simulink model "gtm_aeromodel"  (Simulink 7.2)
settings: Solver=ode45  StartTime=0.0  StopTime=10.0  RelTol=1e-3
undefined symbols (not defined in the file or in its folder): A_BLCG, A_BW, A_CW, A_FSCG, A_FSREF_in, A_SW, A_WLCG, A_WLREF, ALPHA0, bclowb, bclowbx_FMACH, bcmowb, bcmowbx_FHP, bcmowby_FMACH, cda, cdax_FLPDEF, cddr, cddrx_FMACH, cdo, cdox_FLPDEF, cdt1, cdt1x_mach, cdt2, cdt2x_mach, cdto, cdtox_mach, cdwb, cdwbx_FALPHA, cdwby_FMACH, clat, clatfr, clatfrx_FHP, clatfry_FMACH, clatx_mach, clawbfr, clawbfrx_FHP, clawbfry_FMACH, cldefr, cldefrx_FHP, cldefry_FMACH, cldtab, cldtabx_FMACH, clqwb, clqwbfr, clqwbfrx_FHP, clqwbfry_FMACH, clqwbx_mach, cltdd, cltddx_FHP, cltddy_FMACH, clwb, clwbtdd, clwbtddx_FHP, clwbtddy_FMACH, clwbx_FALPHA, clwby_FMACH, clwbzdd, clwbzddx_FHP, clwbzddy_FMACH, clzdd ... (+196)
libraries: model_lib x1
(part 2 of 10)

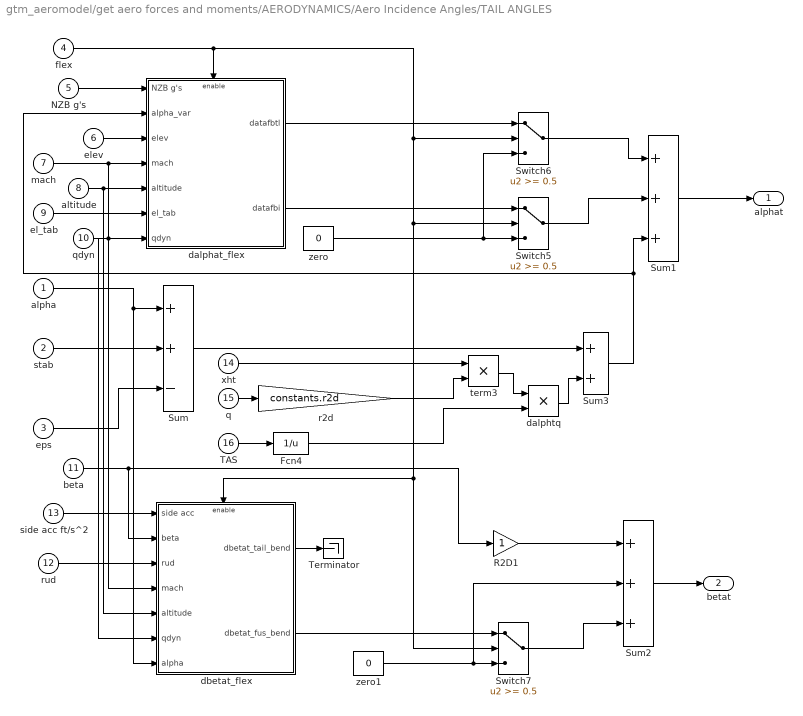
== system gtm_aeromodel/get aero forces and moments/AERODYNAMICS/Aero Incidence Angles/TAIL ANGLES ==
  alpha : Inport  OutDataType=sfix(16)  OutScaling=2^0
  stab : Inport  Port=2  OutDataType=sfix(16)  OutScaling=2^0
  eps : Inport  Port=3  OutDataType=sfix(16)  OutScaling=2^0
  flex : Inport  Port=4  OutDataType=sfix(16)  OutScaling=2^0
  NZB g's : Inport  Port=5  OutDataType=sfix(16)  OutScaling=2^0
  elev : Inport  Port=6  OutDataType=sfix(16)  OutScaling=2^0
  mach : Inport  Port=7  OutDataType=sfix(16)  OutScaling=2^0
  altitude : Inport  Port=8  OutDataType=sfix(16)  OutScaling=2^0
  el_tab : Inport  Port=9  OutDataType=sfix(16)  OutScaling=2^0
  qdyn : Inport  Port=10  OutDataType=sfix(16)  OutScaling=2^0
  beta : Inport  Port=11  OutDataType=sfix(16)  OutScaling=2^0
  rud : Inport  Port=12  OutDataType=sfix(16)  OutScaling=2^0
  side acc ft/s^2 : Inport  Port=13  OutDataType=sfix(16)  OutScaling=2^0
  xht : Inport  Port=14  OutDataType=sfix(16)  OutScaling=2^0
  q : Inport  Port=15  OutDataType=sfix(16)  OutScaling=2^0
  TAS : Inport  Port=16  OutDataType=sfix(16)  OutScaling=2^0
  Fcn4 : Fcn  Expr=1/u
  R2D1 : Gain  ParameterDataType=sfix(16)  ParameterScaling=2^0  OutDataType=sfix(16)  OutScaling=2^0  SaturateOnIntegerOverflow=on  OutDataTypeStr=Inherit: Same as input  ParamDataTypeStr=Inherit: Same as input
  Sum : Sum  Inputs=++-  OutDataType=sfix(16)  OutScaling=2^0  SaturateOnIntegerOverflow=on  InputSameDT=on  OutDataTypeStr=Inherit: Same as first input
  Sum1 : Sum  Inputs=+++  OutDataType=sfix(16)  OutScaling=2^0  SaturateOnIntegerOverflow=on  InputSameDT=on  OutDataTypeStr=Inherit: Same as first input
  Sum2 : Sum  Inputs=+++  OutDataType=sfix(16)  OutScaling=2^0  SaturateOnIntegerOverflow=on  InputSameDT=on  OutDataTypeStr=Inherit: Same as first input
  Sum3 : Sum  OutDataType=sfix(16)  OutScaling=2^0  SaturateOnIntegerOverflow=on  InputSameDT=on  OutDataTypeStr=Inherit: Same as first input
  Switch5 : Switch  Threshold=0.5  SaturateOnIntegerOverflow=on  InputSameDT=on
  Switch6 : Switch  Threshold=0.5  SaturateOnIntegerOverflow=on  InputSameDT=on
  Switch7 : Switch  Threshold=0.5  SaturateOnIntegerOverflow=on  InputSameDT=on
  Terminator : Terminator
  dalphat_flex : Subsystem  TreatAsAtomicUnit=on
  dalphtq : Product  OutDataType=sfix(16)  OutScaling=2^0  SaturateOnIntegerOverflow=on  RndMeth=Zero  InputSameDT=on  OutDataTypeStr=Inherit: Same as first input
  dbetat_flex : Subsystem  TreatAsAtomicUnit=on
  r2d : Gain  Gain=constants.r2d  ParameterDataType=sfix(16)  ParameterScaling=2^0  OutDataType=sfix(16)  OutScaling=2^0  SaturateOnIntegerOverflow=on  OutDataTypeStr=Inherit: Same as input  ParamDataTypeStr=Inherit: Same as input
  term3 : Product  OutDataType=sfix(16)  OutScaling=2^0  SaturateOnIntegerOverflow=on  RndMeth=Zero  InputSameDT=on  OutDataTypeStr=Inherit: Same as first input
  zero : Constant  Value=0  OutDataType=sfix(16)  OutScaling=2^0
  zero1 : Constant  Value=0  OutDataType=sfix(16)  OutScaling=2^0
  alphat : Outport  OutDataType=sfix(16)  OutScaling=2^0
  betat : Outport  Port=2  OutDataType=sfix(16)  OutScaling=2^0
  wires:
  r2d/1 -> term3/2
  q/1 -> r2d/1
  alpha/1 -> Sum/1, dbetat_flex/7(alpha)
  stab/1 -> Sum/2
  eps/1 -> Sum/3
  dalphtq/1 -> Sum3/2
  Switch5/1 -> Sum1/2
  Switch6/1 -> Sum1/1
  R2D1/1 -> Sum2/1
  mach/1 -> dbetat_flex/4(mach), dalphat_flex/4(mach)
  altitude/1 -> dbetat_flex/5(altitude), dalphat_flex/5(altitude)
  qdyn/1 -> dbetat_flex/6(qdyn), dalphat_flex/7(qdyn)
  flex/1 -> dalphat_flex/Enable, dbetat_flex/Enable, Switch7/2, Switch5/2, Switch6/2
  zero/1 -> Switch5/3, Switch6/3
  dalphat_flex/2(datafbi) -> Switch5/1
  NZB g's/1 -> dalphat_flex/1(NZB g's)
  elev/1 -> dalphat_flex/3(elev)
  el_tab/1 -> dalphat_flex/6(el_tab)
  side acc ft/s^2/1 -> dbetat_flex/1("side acc ")
  rud/1 -> dbetat_flex/3(rud)
  beta/1 -> R2D1/1, dbetat_flex/2(beta)
  Sum2/1 -> betat/1
  dbetat_flex/1(dbetat_tail_bend) -> Terminator/1
  xht/1 -> term3/1
  TAS/1 -> Fcn4/1
  term3/1 -> dalphtq/1
  Fcn4/1 -> dalphtq/2
  dalphat_flex/1(datafbtl) -> Switch6/1
  Sum/1 -> Sum3/1
  Sum3/1 -> dalphat_flex/2(alpha_var), Sum1/3
  dbetat_flex/2(dbetat_fus_bend) -> Switch7/1
  Switch7/1 -> Sum2/3
  zero1/1 -> Sum2/2, Switch7/3
  Sum1/1 -> alphat/1

== system gtm_aeromodel/get aero forces and moments/AERODYNAMICS/Force  Coefficients/DRAG  ==
  flex : Inport  OutDataType=sfix(16)  OutScaling=2^0
  ige : Inport  Port=2  OutDataType=sfix(16)  OutScaling=2^0
  hob : Inport  Port=3  OutDataType=sfix(16)  OutScaling=2^0
  alpha : Inport  Port=4  OutDataType=sfix(16)  OutScaling=2^0
  mach : Inport  Port=5  OutDataType=sfix(16)  OutScaling=2^0
  altitude : Inport  Port=6  OutDataType=sfix(16)  OutScaling=2^0
  flap : Inport  Port=7  OutDataType=sfix(16)  OutScaling=2^0
  gear : Inport  Port=8  OutDataType=sfix(16)  OutScaling=2^0
  dsb : Inport  Port=9  OutDataType=sfix(16)  OutScaling=2^0
  dsl : Inport  Port=10  OutDataType=sfix(16)  OutScaling=2^0
  rud : Inport  Port=11  OutDataType=sfix(16)  OutScaling=2^0
  aill : Inport  Port=12  OutDataType=sfix(16)  OutScaling=2^0
  alphat : Inport  Port=13  OutDataType=sfix(16)  OutScaling=2^0
  elev : Inport  Port=14  OutDataType=sfix(16)  OutScaling=2^0
  ailr : Inport  Port=15  OutDataType=sfix(16)  OutScaling=2^0
  dsr : Inport  Port=16  OutDataType=sfix(16)  OutScaling=2^0
  clwb : Inport  Port=17  OutDataType=sfix(16)  OutScaling=2^0
  CDAIL : Subsystem
  CDGE : Subsystem  TreatAsAtomicUnit=on
  CDGEAR : Subsystem
  CDR : Subsystem
  CDSPOIL : Subsystem
  CDTP : Subsystem
  CDWB : Subsystem
  DCDDEL : Subsystem
  Sum1 : Sum  Inputs=+++++  OutDataType=sfix(16)  OutScaling=2^0  SaturateOnIntegerOverflow=on  InputSameDT=on  OutDataTypeStr=Inherit: Same as first input
  Sum8 : Sum  Inputs=++++++++  OutDataType=sfix(16)  OutScaling=2^0  SaturateOnIntegerOverflow=on  InputSameDT=on  OutDataTypeStr=Inherit: Same as first input
  Switch6 : Switch  Threshold=0.5  SaturateOnIntegerOverflow=on  InputSameDT=on
  bcddf : Subsystem  TreatAsAtomicUnit=on
  bcdwb : Subsystem
  constant1 : Constant  Value=0.0  OutDataType=sfix(16)  OutScaling=2^0
  CD8 : Outport  OutDataType=sfix(16)  OutScaling=2^0  InitialOutput=0
  cdtp : Outport  Port=2  OutDataType=sfix(16)  OutScaling=2^0  InitialOutput=0
  dcddel : Outport  Port=3  OutDataType=sfix(16)  OutScaling=2^0  InitialOutput=0
  wires:
  bcddf/1(bcddf) -> Sum8/8
  bcdwb/1(bcdwb_) -> Sum8/7
  DCDDEL/1(dcdde) -> dcddel/1
  CDAIL/1(cdail) -> Sum8/6
  CDTP/1(cdtp) -> cdtp/1
  CDGEAR/1(cdg) -> Sum8/4
  CDR/1(cdrud) -> Sum8/3
  CDSPOIL/3(cd_sp_int_df) -> Sum1/4
  CDSPOIL/2(cd_sb) -> Sum1/3
  CDSPOIL/1(cd_spoil) -> Sum1/2
  CDWB/3(dcdsbfint) -> Sum1/5
  CDWB/2(cd_flap) -> Sum1/1
  CDWB/1(cdwb) -> Sum8/1
  Sum8/1 -> CD8/1
  Sum1/1 -> Sum8/2
  flap/1 -> CDWB/3(flap), CDGEAR/1(flap), CDGE/3(flap), bcddf/1(flap), CDSPOIL/5(flap)
  mach/1 -> CDWB/2(mach), CDR/1(mach), CDTP/1(mach), DCDDEL/3(mach), CDSPOIL/4(mach)
  alpha/1 -> CDWB/1(alpha), CDGEAR/2(alpha), CDGE/2(alpha), CDSPOIL/3(alpha)
  alphat/1 -> CDTP/2(alphat), DCDDEL/2(alphat)
  elev/1 -> DCDDEL/1(elev)
  ailr/1 -> CDAIL/2(ailr)
  hob/1 -> CDGE/1(hob)
  aill/1 -> CDAIL/1(aill)
  constant1/1 -> Switch6/3
  CDGE/1(cdge) -> Switch6/1
  Switch6/1 -> Sum8/5
  ige/1 -> Switch6/2
  rud/1 -> CDR/2(rud)
  gear/1 -> CDGEAR/3(gear)
  dsl/1 -> CDSPOIL/2(dsl)
  dsr/1 -> CDSPOIL/6(dsr)
  altitude/1 -> CDWB/5(altitude)
  flex/1 -> CDWB/4(flex)
  dsb/1 -> CDSPOIL/1(dsb), CDWB/6(dsb)
  clwb/1 -> bcdwb/1(clwb)

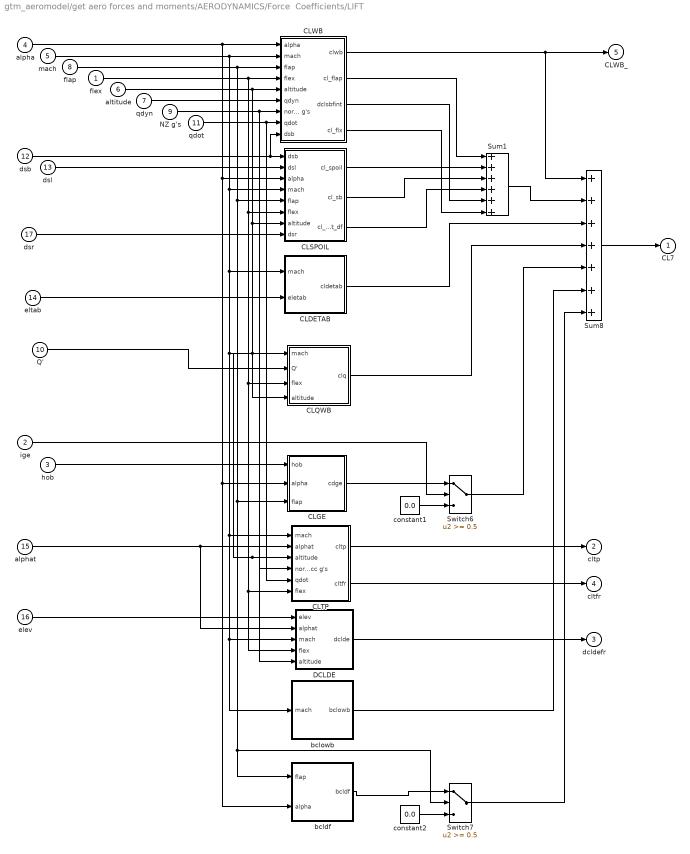
== system gtm_aeromodel/get aero forces and moments/AERODYNAMICS/Force  Coefficients/LIFT ==
  flex : Inport  OutDataType=sfix(16)  OutScaling=2^0
  ige : Inport  Port=2  OutDataType=sfix(16)  OutScaling=2^0
  hob : Inport  Port=3  OutDataType=sfix(16)  OutScaling=2^0
  alpha : Inport  Port=4  OutDataType=sfix(16)  OutScaling=2^0
  mach : Inport  Port=5  OutDataType=sfix(16)  OutScaling=2^0
  altitude : Inport  Port=6  OutDataType=sfix(16)  OutScaling=2^0
  qdyn : Inport  Port=7  OutDataType=sfix(16)  OutScaling=2^0
  flap : Inport  Port=8  OutDataType=sfix(16)  OutScaling=2^0
  NZ g's : Inport  Port=9  OutDataType=sfix(16)  OutScaling=2^0
  Q' : Inport  Port=10  OutDataType=sfix(16)  OutScaling=2^0
  qdot : Inport  Port=11  OutDataType=sfix(16)  OutScaling=2^0
  dsb : Inport  Port=12  OutDataType=sfix(16)  OutScaling=2^0
  dsl : Inport  Port=13  OutDataType=sfix(16)  OutScaling=2^0
  eltab : Inport  Port=14  OutDataType=sfix(16)  OutScaling=2^0
  alphat : Inport  Port=15  OutDataType=sfix(16)  OutScaling=2^0
  elev : Inport  Port=16  OutDataType=sfix(16)  OutScaling=2^0
  dsr : Inport  Port=17  OutDataType=sfix(16)  OutScaling=2^0
  CLDETAB : Subsystem
  CLGE : Subsystem  TreatAsAtomicUnit=on
  CLQWB : Subsystem
  CLSPOIL : Subsystem
  CLTP : Subsystem
  CLWB : Subsystem
  DCLDE : Subsystem
  Sum1 : Sum  Inputs=++++++  OutDataType=sfix(16)  OutScaling=2^0  SaturateOnIntegerOverflow=on  InputSameDT=on  OutDataTypeStr=Inherit: Same as first input
  Sum8 : Sum  Inputs=+++++++  OutDataType=sfix(16)  OutScaling=2^0  SaturateOnIntegerOverflow=on  InputSameDT=on  OutDataTypeStr=Inherit: Same as first input
  Switch6 : Switch  Threshold=0.5  SaturateOnIntegerOverflow=on  InputSameDT=on
  Switch7 : Switch  Threshold=0.5  SaturateOnIntegerOverflow=on  InputSameDT=on
  bcldf : Subsystem  TreatAsAtomicUnit=on
  bclowb : Subsystem
  constant1 : Constant  Value=0.0  OutDataType=sfix(16)  OutScaling=2^0
  constant2 : Constant  Value=0.0  OutDataType=sfix(16)  OutScaling=2^0
  CL7 : Outport  OutDataType=sfix(16)  OutScaling=2^0  InitialOutput=0
  cltp : Outport  Port=2  OutDataType=sfix(16)  OutScaling=2^0  InitialOutput=0
  dcldefr : Outport  Port=3  OutDataType=sfix(16)  OutScaling=2^0  InitialOutput=0
  cltfr : Outport  Port=4  OutDataType=sfix(16)  OutScaling=2^0  InitialOutput=0
  CLWB_ : Outport  Port=5  OutDataType=sfix(16)  OutScaling=2^0  InitialOutput=0
  wires:
  CLWB/4(cl_flx) -> Sum1/6
  CLWB/1(clwb) -> CLWB_/1, Sum8/1
  alpha/1 -> CLSPOIL/3(alpha), CLGE/2(alpha), bcldf/2(alpha), CLWB/1(alpha)
  mach/1 -> CLSPOIL/4(mach), bclowb/1(mach), DCLDE/3(mach), CLTP/1(mach), CLQWB/1(mach), CLDETAB/1(mach), CLWB/2(mach)
  flap/1 -> CLSPOIL/5(flap), CLGE/3(flap), Switch7/2, bcldf/1(flap), CLWB/3(flap)
  altitude/1 -> DCLDE/5(altitude), CLTP/3(altitude), CLQWB/4(altitude), CLSPOIL/7(altitude), CLWB/5(altitude)
  qdot/1 -> CLTP/5(qdot), CLWB/8(qdot)
  NZ g's/1 -> CLTP/4(norm acc g's), CLWB/7(norm acc g's)
  qdyn/1 -> CLWB/6(qdyn)
  flex/1 -> CLQWB/3(flex), DCLDE/4(flex), CLTP/6(flex), CLSPOIL/6(flex), CLWB/4(flex)
  Switch7/1 -> Sum8/7
  bclowb/1(bclowb) -> Sum8/6
  CLTP/1(cltp) -> cltp/1
  DCLDE/1(dclde) -> dcldefr/1
  CLTP/2(cltfr) -> cltfr/1
  CLQWB/1(clq) -> Sum8/4
  CLSPOIL/3(cl_sp_int_df) -> Sum1/4
  CLDETAB/1(cldetab) -> Sum8/3
  CLSPOIL/2(cl_sb) -> Sum1/3
  CLSPOIL/1(cl_spoil) -> Sum1/2
  CLWB/3(dclsbfint) -> Sum1/5
  CLWB/2(cl_flap) -> Sum1/1
  dsb/1 -> CLWB/9(dsb), CLSPOIL/1(dsb)
  dsr/1 -> CLSPOIL/8(dsr)
  hob/1 -> CLGE/1(hob)
  ige/1 -> Switch6/2
  CLGE/1(cdge) -> Switch6/1
  Switch6/1 -> Sum8/5
  elev/1 -> DCLDE/1(elev)
  alphat/1 -> DCLDE/2(alphat), CLTP/2(alphat)
  eltab/1 -> CLDETAB/2(eletab)
  dsl/1 -> CLSPOIL/2(dsl)
  Sum8/1 -> CL7/1
  Sum1/1 -> Sum8/2
  constant1/1 -> Switch6/3
  constant2/1 -> Switch7/3
  bcldf/1(bcldf) -> Switch7/1
  Q'/1 -> CLQWB/2(Q')

== system gtm_aeromodel/get aero forces and moments/AERODYNAMICS/Force  Coefficients/SIDE ==
  note: dcyt
  flex : Inport  OutDataType=sfix(16)  OutScaling=2^0
  alpha : Inport  Port=2  OutDataType=sfix(16)  OutScaling=2^0
  mach : Inport  Port=3  OutDataType=sfix(16)  OutScaling=2^0
  altitude : Inport  Port=4  OutDataType=sfix(16)  OutScaling=2^0
  flap : Inport  Port=5  OutDataType=sfix(16)  OutScaling=2^0
  gear : Inport  Port=6  OutDataType=sfix(16)  OutScaling=2^0
  dsb : Inport  Port=7  OutDataType=sfix(16)  OutScaling=2^0
  dsl : Inport  Port=8  OutDataType=sfix(16)  OutScaling=2^0
  rud : Inport  Port=9  OutDataType=sfix(16)  OutScaling=2^0
  beta : Inport  Port=10  OutDataType=sfix(16)  OutScaling=2^0
  betat : Inport  Port=11  OutDataType=sfix(16)  OutScaling=2^0
  p_prime : Inport  Port=12  OutDataType=sfix(16)  OutScaling=2^0
  r_prime : Inport  Port=13  OutDataType=sfix(16)  OutScaling=2^0
  dsr : Inport  Port=14  OutDataType=sfix(16)  OutScaling=2^0
  " " : Product  Inputs=3  OutDataType=sfix(16)  OutScaling=2^0  SaturateOnIntegerOverflow=on  RndMeth=Zero  InputSameDT=on  OutDataTypeStr=Inherit: Same as first input
  CYBWB : Subsystem
  CYGEAR : Subsystem
  CYP : Subsystem
  CYR : Subsystem
  CYRUD : Subsystem
  CYSPOIL : Subsystem
  Sum8 : Sum  Inputs=+++++++  OutDataType=sfix(16)  OutScaling=2^0  SaturateOnIntegerOverflow=on  InputSameDT=on  OutDataTypeStr=Inherit: Same as first input
  Switch5 : Switch  Threshold=0.1  SaturateOnIntegerOverflow=on  InputSameDT=on
  TAIL : Subsystem
  constant : Constant  OutDataType=sfix(16)  OutScaling=2^0
  cybwb : Product  Inputs=3  OutDataType=sfix(16)  OutScaling=2^0  SaturateOnIntegerOverflow=on  RndMeth=Zero  InputSameDT=on  OutDataTypeStr=Inherit: Same as first input
  CYS : Outport  OutDataType=sfix(16)  OutScaling=2^0  InitialOutput=0
  wires:
  CYGEAR/1(cdg) -> Sum8/7
  CYR/1(dcyrhat) -> Sum8/6
  CYP/1(dcyphat) -> Sum8/5
  CYSPOIL/1(cy_spoil) -> Sum8/3
  " "/1 -> Sum8/2
  cybwb/1 -> Sum8/1
  beta/1 -> CYGEAR/4(beta), cybwb/3
  gear/1 -> CYGEAR/3(gear)
  r_prime/1 -> CYR/5(r_prime)
  p_prime/1 -> CYP/5(p_prime)
  altitude/1 -> CYR/3(altitude), CYP/3(altitude), CYRUD/3(altitude), CYBWB/5(altitude)
  rud/1 -> CYRUD/2(rud)
  flap/1 -> CYGEAR/1(flap), CYSPOIL/5(flap), CYBWB/3(flap)
  TAIL/1(cyb_ht_vt) -> " "/2
  alpha/1 -> CYGEAR/2(alpha), CYR/2(alpha), CYP/2(alpha), CYSPOIL/3(alpha), TAIL/2(alpha), CYBWB/1(alpha)
  mach/1 -> CYR/1(mach), CYP/1(mach), CYRUD/1(mach), CYSPOIL/4(mach), TAIL/1(mach), CYBWB/2(mach)
  flex/1 -> CYR/4(flex), CYP/4(flex), CYRUD/4(flex), Switch5/2, CYBWB/4(flex)
  betat/1 -> " "/3
  Switch5/1 -> " "/1, cybwb/2
  CYBWB/2(cybfr) -> Switch5/1
  constant/1 -> Switch5/3
  Sum8/1 -> CYS/1
  dsb/1 -> CYSPOIL/1(dsb)
  dsl/1 -> CYSPOIL/2(dsl)
  dsr/1 -> CYSPOIL/6(dsr)
  CYBWB/1(cywb+fl) -> cybwb/1
  CYRUD/1(cyrud) -> Sum8/4

== system gtm_aeromodel/get aero forces and moments/AERODYNAMICS/Moment Coefficients/PITCH ==
  flex : Inport  OutDataType=sfix(16)  OutScaling=2^0
  alpha : Inport  Port=2  OutDataType=sfix(16)  OutScaling=2^0
  mach : Inport  Port=3  OutDataType=sfix(16)  OutScaling=2^0
  altitude : Inport  Port=4  OutDataType=sfix(16)  OutScaling=2^0
  qdyn : Inport  Port=5  OutDataType=sfix(16)  OutScaling=2^0
  flap : Inport  Port=6  OutDataType=sfix(16)  OutScaling=2^0
  dsb : Inport  Port=7  OutDataType=sfix(16)  OutScaling=2^0
  dsl : Inport  Port=8  OutDataType=sfix(16)  OutScaling=2^0
  NZ g's : Inport  Port=9  OutDataType=sfix(16)  OutScaling=2^0
  qdot : Inport  Port=10  OutDataType=sfix(16)  OutScaling=2^0
  qhat : Inport  Port=11  OutDataType=sfix(16)  OutScaling=2^0
  eltab : Inport  Port=12  OutDataType=sfix(16)  OutScaling=2^0
  alphat : Inport  Port=13  OutDataType=sfix(16)  OutScaling=2^0
  elev : Inport  Port=14  OutDataType=sfix(16)  OutScaling=2^0
  dsr : Inport  Port=15  OutDataType=sfix(16)  OutScaling=2^0
  BCMOWB : Subsystem
  CMQWB : Subsystem
  CMSPOIL : Subsystem
  CMT : Subsystem
  CMTAB : Subsystem
  CMWB : Subsystem
  DCMDE : Subsystem
  Look-Up Table : Lookup  InputValues="[0  200  350]"  Table=[1 0.76 0.7]  OutDataType=sfix(16)  OutScaling=2^0  SaturateOnIntegerOverflow=on
  Product : Product  OutDataType=sfix(16)  OutScaling=2^0  SaturateOnIntegerOverflow=on  RndMeth=Zero  InputSameDT=on  OutDataTypeStr=Inherit: Same as first input
  Sum1 : Sum  Inputs=++++++  OutDataType=sfix(16)  OutScaling=2^0  SaturateOnIntegerOverflow=on  InputSameDT=on  OutDataTypeStr=Inherit: Same as first input
  Sum8 : Sum  Inputs=++++++++  OutDataType=sfix(16)  OutScaling=2^0  SaturateOnIntegerOverflow=on  InputSameDT=on  OutDataTypeStr=Inherit: Same as first input
  bcmdf : Subsystem  TreatAsAtomicUnit=on
  CMS : Outport  OutDataType=sfix(16)  OutScaling=2^0  InitialOutput=0
  CMDE : Outport  Port=2  OutDataType=sfix(16)  OutScaling=2^0  InitialOutput=0
  wires:
  bcmdf/1(bcmdf) -> Sum8/8
  BCMOWB/1(bcmowb) -> Sum8/7
  CMT/1(cmt) -> Sum8/5
  CMQWB/1(dcmqwb) -> Sum8/4
  CMTAB/1(cmtab) -> Sum8/3
  CMSPOIL/3(dcmspfint) -> Sum1/4
  CMSPOIL/2(cm_sb) -> Sum1/3
  CMSPOIL/1(cm_spoil) -> Sum1/2
  CMWB/2(cm_flap) -> Sum1/1
  CMWB/3(dcmsbfint) -> Sum1/5
  CMWB/1(cmwb) -> Sum8/1
  Sum8/1 -> CMS/1
  Sum1/1 -> Sum8/2
  flex/1 -> CMSPOIL/6(flex), CMQWB/3(flex), CMT/6(flex), DCMDE/4(flex), CMTAB/4(flex), CMWB/4(flex)
  qdyn/1 -> CMWB/6(qdyn), Look-Up Table/1
  flap/1 -> CMWB/3(flap), CMSPOIL/5(flap), bcmdf/1(flap)
  mach/1 -> CMTAB/1(mach), CMQWB/1(mach), CMT/1(mach), DCMDE/3(mach), BCMOWB/1(mach), CMSPOIL/4(mach), CMWB/2(mach)
  alpha/1 -> CMWB/1(alpha), CMSPOIL/3(alpha), bcmdf/2(alpha)
  dsl/1 -> CMSPOIL/2(dsl)
  qdot/1 -> CMWB/8(qdot), CMT/5(qdot)
  elev/1 -> DCMDE/1(elev)
  qhat/1 -> CMQWB/2(qhat)
  eltab/1 -> CMTAB/2(eletab)
  dsb/1 -> CMSPOIL/1(dsb), CMWB/9(dsb)
  dsr/1 -> CMSPOIL/8(dsr)
  NZ g's/1 -> CMWB/7(norm acc g's), CMT/4(norm acc g's)
  altitude/1 -> CMWB/5(altitude), CMSPOIL/7(altitude), CMTAB/3(alt), CMQWB/4(altitude), CMT/3(altitude), DCMDE/5(altitude), BCMOWB/2(altitude)
  CMWB/4(cm_flx) -> Sum1/6
  alphat/1 -> CMT/2(alphat), DCMDE/2(alphat)
  Look-Up Table/1 -> Product/2
  DCMDE/1(dcmde) -> Product/1
  Product/1 -> CMDE/1, Sum8/6

== system gtm_aeromodel/get aero forces and moments/AERODYNAMICS/Moment Coefficients/ROLL ==
  note: dclt
  flex : Inport  OutDataType=sfix(16)  OutScaling=2^0
  alpha : Inport  Port=2  OutDataType=sfix(16)  OutScaling=2^0
  mach : Inport  Port=3  OutDataType=sfix(16)  OutScaling=2^0
  altitude : Inport  Port=4  OutDataType=sfix(16)  OutScaling=2^0
  flap : Inport  Port=5  OutDataType=sfix(16)  OutScaling=2^0
  gear : Inport  Port=6  OutDataType=sfix(16)  OutScaling=2^0
  dsb : Inport  Port=7  OutDataType=sfix(16)  OutScaling=2^0
  dsl : Inport  Port=8  OutDataType=sfix(16)  OutScaling=2^0
  rud : Inport  Port=9  OutDataType=sfix(16)  OutScaling=2^0
  beta : Inport  Port=10  OutDataType=sfix(16)  OutScaling=2^0
  betat : Inport  Port=11  OutDataType=sfix(16)  OutScaling=2^0
  phat : Inport  Port=12  OutDataType=sfix(16)  OutScaling=2^0
  rhat : Inport  Port=13  OutDataType=sfix(16)  OutScaling=2^0
  aill : Inport  Port=14  OutDataType=sfix(16)  OutScaling=2^0
  TAS : Inport  Port=15  OutDataType=sfix(16)  OutScaling=2^0
  ailr : Inport  Port=16  OutDataType=sfix(16)  OutScaling=2^0
  dsr : Inport  Port=17  OutDataType=sfix(16)  OutScaling=2^0
  dadot : Inport  Port=18  OutDataType=sfix(16)  OutScaling=2^0
  " " : Product  Inputs=3  OutDataType=sfix(16)  OutScaling=2^0  SaturateOnIntegerOverflow=on  RndMeth=Zero  InputSameDT=on  OutDataTypeStr=Inherit: Same as first input
  CRAIL : Subsystem
  CRBWB : Subsystem
  CRGEAR : Subsystem
  CRP : Subsystem
  CRR : Subsystem
  CRRUD : Subsystem
  CRSPOIL : Subsystem
  R2D3 : Gain  ParameterDataType=sfix(16)  ParameterScaling=2^0  OutDataType=sfix(16)  OutScaling=2^0  SaturateOnIntegerOverflow=on  OutDataTypeStr=Inherit: Same as input  ParamDataTypeStr=Inherit: Same as input
  R2D4 : Gain  ParameterDataType=sfix(16)  ParameterScaling=2^0  OutDataType=sfix(16)  OutScaling=2^0  SaturateOnIntegerOverflow=on  OutDataTypeStr=Inherit: Same as input  ParamDataTypeStr=Inherit: Same as input
  Sum8 : Sum  Inputs=++++++++  OutDataType=sfix(16)  OutScaling=2^0  SaturateOnIntegerOverflow=on  InputSameDT=on  OutDataTypeStr=Inherit: Same as first input
  Switch5 : Switch  Threshold=0.1  SaturateOnIntegerOverflow=on  InputSameDT=on
  TAIL : Subsystem
  constant : Constant  OutDataType=sfix(16)  OutScaling=2^0
  crbwb : Product  Inputs=3  OutDataType=sfix(16)  OutScaling=2^0  SaturateOnIntegerOverflow=on  RndMeth=Zero  InputSameDT=on  OutDataTypeStr=Inherit: Same as first input
  CRS : Outport  OutDataType=sfix(16)  OutScaling=2^0  InitialOutput=0
  wires:
  CRAIL/1(crail) -> Sum8/8
  CRGEAR/1(crg) -> Sum8/7
  CRR/1(dcrrhat) -> Sum8/6
  CRP/1(dcrphat) -> Sum8/5
  CRRUD/1(crrud) -> Sum8/4
  CRSPOIL/1(cr_spoil) -> Sum8/3
  " "/1 -> Sum8/2
  crbwb/1 -> Sum8/1
  R2D4/1 -> CRR/5(rhat)
  rhat/1 -> R2D4/1
  R2D3/1 -> CRP/5(phat)
  phat/1 -> R2D3/1
  dadot/1 -> CRAIL/9(dadot)
  ailr/1 -> CRAIL/8(ailr)
  TAS/1 -> CRAIL/7(TAS)
  aill/1 -> CRAIL/1(aill)
  Sum8/1 -> CRS/1
  CRBWB/1(crbwb_fl) -> crbwb/1
  constant/1 -> Switch5/3
  CRBWB/2(crbfr) -> Switch5/1
  Switch5/1 -> " "/1, crbwb/2
  betat/1 -> " "/3
  flex/1 -> CRBWB/4(flex), CRSPOIL/7(flex), CRRUD/4(flex), CRAIL/2(flex), CRR/4(flex), CRP/4(flex), Switch5/2
  mach/1 -> CRBWB/2(mach), TAIL/1(mach), CRAIL/3(mach), CRR/1(mach), CRP/1(mach), CRRUD/5(mach), CRSPOIL/4(mach)
  alpha/1 -> CRBWB/1(alpha), TAIL/2(alpha), CRAIL/4(alpha), CRR/2(alpha), CRP/2(alpha), CRRUD/1(alpha), CRSPOIL/3(alpha)
  TAIL/1(crt) -> " "/2
  dsb/1 -> CRSPOIL/1(dsb)
  dsl/1 -> CRSPOIL/2(dsl)
  flap/1 -> CRBWB/3(flap), CRAIL/5(flap), CRGEAR/1(flap), CRSPOIL/5(flap)
  rud/1 -> CRRUD/2(rud)
  altitude/1 -> CRSPOIL/6(altitude), CRAIL/6(altitude), CRR/3(altitude), CRP/3(altitude), CRRUD/3(altitude), CRBWB/5(altitude)
  gear/1 -> CRGEAR/2(gear)
  beta/1 -> crbwb/3, CRGEAR/3(beta)
  dsr/1 -> CRSPOIL/8(dsr)

== system gtm_aeromodel/get aero forces and moments/AERODYNAMICS/Moment Coefficients/YAW ==
  note: dcnt
  flex : Inport  OutDataType=sfix(16)  OutScaling=2^0
  alpha : Inport  Port=2  OutDataType=sfix(16)  OutScaling=2^0
  mach : Inport  Port=3  OutDataType=sfix(16)  OutScaling=2^0
  altitude : Inport  Port=4  OutDataType=sfix(16)  OutScaling=2^0
  flap : Inport  Port=5  OutDataType=sfix(16)  OutScaling=2^0
  gear : Inport  Port=6  OutDataType=sfix(16)  OutScaling=2^0
  dsb : Inport  Port=7  OutDataType=sfix(16)  OutScaling=2^0
  dsl : Inport  Port=8  OutDataType=sfix(16)  OutScaling=2^0
  rud : Inport  Port=9  OutDataType=sfix(16)  OutScaling=2^0
  beta : Inport  Port=10  OutDataType=sfix(16)  OutScaling=2^0
  betat : Inport  Port=11  OutDataType=sfix(16)  OutScaling=2^0
  phat : Inport  Port=12  OutDataType=sfix(16)  OutScaling=2^0
  rhat : Inport  Port=13  OutDataType=sfix(16)  OutScaling=2^0
  dsr : Inport  Port=14  OutDataType=sfix(16)  OutScaling=2^0
  " " : Product  Inputs=3  OutDataType=sfix(16)  OutScaling=2^0  SaturateOnIntegerOverflow=on  RndMeth=Zero  InputSameDT=on  OutDataTypeStr=Inherit: Same as first input
  CNBWB : Subsystem
  CNGEAR : Subsystem
  CNP : Subsystem
  CNR : Subsystem
  CNRUD : Subsystem
  CNSPOIL : Subsystem
  CNT : Subsystem
  Gain : Gain  Gain=1.3  ParameterDataType=sfix(16)  ParameterScaling=2^0  OutDataType=sfix(16)  OutScaling=2^0  SaturateOnIntegerOverflow=on  OutDataTypeStr=Inherit: Same as input  ParamDataTypeStr=Inherit: Same as input
  R2D3 : Gain  ParameterDataType=sfix(16)  ParameterScaling=2^0  OutDataType=sfix(16)  OutScaling=2^0  SaturateOnIntegerOverflow=on  OutDataTypeStr=Inherit: Same as input  ParamDataTypeStr=Inherit: Same as input
  R2D4 : Gain  ParameterDataType=sfix(16)  ParameterScaling=2^0  OutDataType=sfix(16)  OutScaling=2^0  SaturateOnIntegerOverflow=on  OutDataTypeStr=Inherit: Same as input  ParamDataTypeStr=Inherit: Same as input
  Sum8 : Sum  Inputs=+++++++  OutDataType=sfix(16)  OutScaling=2^0  SaturateOnIntegerOverflow=on  InputSameDT=on  OutDataTypeStr=Inherit: Same as first input
  Switch5 : Switch  Threshold=0.1  SaturateOnIntegerOverflow=on  InputSameDT=on
  cnbwb : Product  Inputs=3  OutDataType=sfix(16)  OutScaling=2^0  SaturateOnIntegerOverflow=on  RndMeth=Zero  InputSameDT=on  OutDataTypeStr=Inherit: Same as first input
  constant : Constant  OutDataType=sfix(16)  OutScaling=2^0
  CNS : Outport  OutDataType=sfix(16)  OutScaling=2^0  InitialOutput=0
  wires:
  altitude/1 -> CNBWB/5(altitude), CNR/3(altitude), CNP/3(altitude), CNRUD/2(altitude)
  flap/1 -> CNBWB/3(flap), CNGEAR/1(flap), CNSPOIL/5(flap)
  alpha/1 -> CNR/2(alpha), CNP/2(alpha), CNSPOIL/3(alpha), CNT/2(alpha), CNBWB/1(alpha)
  mach/1 -> CNT/1(mach), CNSPOIL/4(mach), CNRUD/4(mach), CNR/1(mach), CNP/1(mach), CNBWB/2(mach)
  flex/1 -> Switch5/2, CNR/4(flex), CNP/4(flex), CNRUD/3(flex), CNBWB/4(flex)
  R2D4/1 -> CNR/5(rhat)
  rhat/1 -> R2D4/1
  R2D3/1 -> CNP/5(phat)
  phat/1 -> R2D3/1
  dsr/1 -> CNSPOIL/6(dsr)
  beta/1 -> CNGEAR/3(beta), cnbwb/3
  CNSPOIL/1(cn_spoil) -> Sum8/3
  dsl/1 -> CNSPOIL/2(dsl)
  dsb/1 -> CNSPOIL/1(dsb)
  " "/1 -> Gain/1
  CNT/1(cnt) -> " "/2
  betat/1 -> " "/3
  Switch5/1 -> " "/1, cnbwb/2
  CNBWB/2(cnbfr) -> Switch5/1
  constant/1 -> Switch5/3
  CNBWB/1(cnbwb) -> cnbwb/1
  Sum8/1 -> CNS/1
  cnbwb/1 -> Sum8/1
  CNGEAR/1(cng) -> Sum8/7
  gear/1 -> CNGEAR/2(gear)
  CNR/1(dcnrhat) -> Sum8/6
  CNP/1(dcnphat) -> Sum8/5
  CNRUD/1(cnrud) -> Sum8/4
  rud/1 -> CNRUD/1(rud)
  Gain/1 -> Sum8/2

== system gtm_aeromodel/get aero forces and moments/AERODYNAMICS/XFORMATION of  AERO FORCES and MOMENTS   to cg centered body axis/CP2CG ==
  note: YCGBR
  note: ZCGCR
  note: ZCGBR
  note: XCGCR
  note: XCGBR
  note: Model Text: CP2CG      Rev.: -
      | Description: Center of Pressure to C.G. Axis Transformation
      | Program: RAYTHEON HAWKER HORIZON
      | PCR No.: N/A    Next Block: AEROLOAD
      |   Written By: G. CHAN    Date: 12-01-98
  note: CRcg = CRb - Cy*Zcg_b - Cz*Ycg_b
      |
      | CMcg = CM + Cx*Zcg_c - Cz*Xcg_c
      |
      | CNcg = CNb + Cy*Xcg_b + Cx*Ycg_b
  Cx Cy Cz : Inport  OutDataType=sfix(16)  OutScaling=2^0
  CRb CMb CNb : Inport  Port=2  OutDataType=sfix(16)  OutScaling=2^0
  FScg WLcg BLcg : Inport  Port=3  OutDataType=sfix(16)  OutScaling=2^0
  Constant20 : Constant  Value=A_FSREF_in  OutDataType=sfix(16)  OutScaling=2^0
  Constant22 : Constant  Value=A_WLREF  OutDataType=sfix(16)  OutScaling=2^0
  Constant24 : Constant  Value=A_BW  OutDataType=sfix(16)  OutScaling=2^0
  Constant25 : Constant  Value=A_CW  OutDataType=sfix(16)  OutScaling=2^0
  Demux : Demux  Outputs=3
  Demux1 : Demux  Outputs=3
  Demux2 : Demux  Outputs=3
  Gain : Gain  Gain=1/12  ParameterDataType=sfix(16)  ParameterScaling=2^0  OutDataType=sfix(16)  OutScaling=2^0  SaturateOnIntegerOverflow=on  OutDataTypeStr=Inherit: Same as input  ParamDataTypeStr=Inherit: Same as input
  Gain1 : Gain  Gain=1/12  ParameterDataType=sfix(16)  ParameterScaling=2^0  OutDataType=sfix(16)  OutScaling=2^0  SaturateOnIntegerOverflow=on  OutDataTypeStr=Inherit: Same as input  ParamDataTypeStr=Inherit: Same as input
  Gain2 : Gain  Gain=1/12  ParameterDataType=sfix(16)  ParameterScaling=2^0  OutDataType=sfix(16)  OutScaling=2^0  SaturateOnIntegerOverflow=on  OutDataTypeStr=Inherit: Same as input  ParamDataTypeStr=Inherit: Same as input
  Mux1 : Mux  Inputs=3
  Product{16..21} (6 alike) : Product  OutDataType=sfix(16)  OutScaling=2^0  SaturateOnIntegerOverflow=on  RndMeth=Zero  InputSameDT=on  OutDataTypeStr=Inherit: Same as first input
  Product22 : Product  Inputs=*/  OutDataType=sfix(16)  OutScaling=2^0  SaturateOnIntegerOverflow=on  RndMeth=Zero  InputSameDT=on  OutDataTypeStr=Inherit: Same as first input
  Product23 : Product  Inputs=*/  OutDataType=sfix(16)  OutScaling=2^0  SaturateOnIntegerOverflow=on  RndMeth=Zero  InputSameDT=on  OutDataTypeStr=Inherit: Same as first input
  Product24 : Product  Inputs=/*  OutDataType=sfix(16)  OutScaling=2^0  SaturateOnIntegerOverflow=on  RndMeth=Zero  InputSameDT=on  OutDataTypeStr=Inherit: Same as first input
  Product25 : Product  Inputs=/*  OutDataType=sfix(16)  OutScaling=2^0  SaturateOnIntegerOverflow=on  RndMeth=Zero  InputSameDT=on  OutDataTypeStr=Inherit: Same as first input
  Product26 : Product  Inputs=/*  OutDataType=sfix(16)  OutScaling=2^0  SaturateOnIntegerOverflow=on  RndMeth=Zero  InputSameDT=on  OutDataTypeStr=Inherit: Same as first input
  Sum : Sum  Inputs=+-  OutDataType=sfix(16)  OutScaling=2^0  SaturateOnIntegerOverflow=on  InputSameDT=on  OutDataTypeStr=Inherit: Same as first input
  Sum1 : Sum  Inputs=+-  OutDataType=sfix(16)  OutScaling=2^0  SaturateOnIntegerOverflow=on  InputSameDT=on  OutDataTypeStr=Inherit: Same as first input
  Sum10 : Sum  Inputs=+--  OutDataType=sfix(16)  OutScaling=2^0  SaturateOnIntegerOverflow=on  InputSameDT=on  OutDataTypeStr=Inherit: Same as first input
  Sum11 : Sum  Inputs=++-  OutDataType=sfix(16)  OutScaling=2^0  SaturateOnIntegerOverflow=on  InputSameDT=on  OutDataTypeStr=Inherit: Same as first input
  Sum12 : Sum  Inputs=+++  OutDataType=sfix(16)  OutScaling=2^0  SaturateOnIntegerOverflow=on  InputSameDT=on  OutDataTypeStr=Inherit: Same as first input
  CRcg CMcg CNcg : Outport  OutDataType=sfix(16)  OutScaling=2^0  InitialOutput=0
  wires:
  Product26/1 -> Product21/2, Product17/2
  Product22/1 -> Product20/2
  Product23/1 -> Product18/2
  Product25/1 -> Product19/2
  Product24/1 -> Product16/2
  Constant20/1 -> Sum/2
  Sum1/1 -> Gain1/1
  Constant22/1 -> Sum1/2
  Gain2/1 -> Product26/2
  Gain1/1 -> Product25/2, Product24/2
  Constant25/1 -> Product25/1, Product23/2
  Constant24/1 -> Product24/1, Product26/1, Product22/2
  Demux/1 -> Product21/1, Product19/1
  Demux/2 -> Product20/1, Product16/1
  Demux/3 -> Product18/1, Product17/1
  Demux2/3 -> Sum12/1
  Demux2/2 -> Sum11/1
  Demux2/1 -> Sum10/1
  Sum12/1 -> Mux1/3
  Sum11/1 -> Mux1/2
  Sum10/1 -> Mux1/1
  Product21/1 -> Sum12/3
  Product20/1 -> Sum12/2
  Product19/1 -> Sum11/2
  Product18/1 -> Sum11/3
  Product17/1 -> Sum10/3
  Product16/1 -> Sum10/2
  Cx Cy Cz/1 -> Demux/1
  Mux1/1 -> CRcg CMcg CNcg/1
  CRb CMb CNb/1 -> Demux2/1
  Gain/1 -> Product23/1, Product22/1
  Sum/1 -> Gain/1
  Demux1/1 -> Sum/1
  FScg WLcg BLcg/1 -> Demux1/1
  Demux1/2 -> Sum1/1
  Demux1/3 -> Gain2/1

== system gtm_aeromodel/get aero forces and moments/AERODYNAMICS/XFORMATION of  AERO FORCES and MOMENTS   to cg centered body axis/DIMENSION ==
  Vtas EASkts Mach Qdyn CASkts : Inport  OutDataType=sfix(16)  OutScaling=2^0
  Cx Cy Cz : Inport  Port=2  OutDataType=sfix(16)  OutScaling=2^0
  CRcg CMcg CNcg : Inport  Port=3  OutDataType=sfix(16)  OutScaling=2^0
  Constant : Constant  Value=A_SW  OutDataType=sfix(16)  OutScaling=2^0
  Constant1 : Constant  Value=A_BW  OutDataType=sfix(16)  OutScaling=2^0
  Constant2 : Constant  Value=A_CW  OutDataType=sfix(16)  OutScaling=2^0
  Demux : Demux  Outputs=3
  Demux2 : Demux  Outputs=3
  Fcn2 : Fcn  Expr=u[4]
  Mux : Mux  Inputs=3
  Mux1 : Mux  Inputs=3
  Product{,1..8} (9 alike) : Product  OutDataType=sfix(16)  OutScaling=2^0  SaturateOnIntegerOverflow=on  RndMeth=Zero  InputSameDT=on  OutDataTypeStr=Inherit: Same as first input
  Xa Ya Za : Outport  OutDataType=sfix(16)  OutScaling=2^0  InitialOutput=0
  La Ma Na : Outport  Port=2  OutDataType=sfix(16)  OutScaling=2^0  InitialOutput=0
  wires:
  Demux2/3 -> Product4/2
  Demux2/1 -> Product6/2
  Product4/1 -> Mux1/3
  Product5/1 -> Mux1/2
  Product6/1 -> Mux1/1
  Product/1 -> Mux/1
  Product2/1 -> Mux/2
  Product3/1 -> Mux/3
  Demux2/2 -> Product5/2
  Product8/1 -> Product5/1
  Fcn2/1 -> Product1/2
  Constant1/1 -> Product7/1
  Constant2/1 -> Product8/1
  Product7/1 -> Product6/1, Product4/1
  Product1/1 -> Product/1, Product2/1, Product3/1, Product8/2, Product7/2
  Demux/1 -> Product/2
  Demux/2 -> Product2/2
  Demux/3 -> Product3/2
  Vtas EASkts Mach Qdyn CASkts/1 -> Fcn2/1
  Mux/1 -> Xa Ya Za/1
  Cx Cy Cz/1 -> Demux/1
  Mux1/1 -> La Ma Na/1
  CRcg CMcg CNcg/1 -> Demux2/1
  Constant/1 -> Product1/1

== system gtm_aeromodel/get aero forces and moments/AERODYNAMICS/XFORMATION of  AERO FORCES and MOMENTS   to cg centered body axis/STAB2BODY ==
  note: Crb
  note: Cnb
  note: Cx =  Cls*sin(alpha)-Cds*cos(alpha
      | Cy =  Cys
      | Cz = -Cls*cos(alpha)-Cds*sin(alpha)
  note: Crb = Crs*cos(alpha) - Cns*sin(alpha)
      | Cnb = Crs*sin(alpha) +Cns*cos(alpha)
      | Cmb = Cms
  alpha beta alpha_dot beta_dot : Inport  OutDataType=sfix(16)  OutScaling=2^0
  CL CD CY : Inport  Port=2  OutDataType=sfix(16)  OutScaling=2^0
  CR CM CN : Inport  Port=3  OutDataType=sfix(16)  OutScaling=2^0
  Demux : Demux  Outputs=3
  Demux2 : Demux  Outputs=3
  Fcn1 : Fcn  Expr=u[1]
  Gain2 : Gain  Gain=pi/180  ParameterDataType=sfix(16)  ParameterScaling=2^0  OutDataType=sfix(16)  OutScaling=2^0  SaturateOnIntegerOverflow=on  OutDataTypeStr=Inherit: Same as input  ParamDataTypeStr=Inherit: Same as input
  Mux : Mux  Inputs=3
  Mux1 : Mux  Inputs=3
  Product{,9..15} (8 alike) : Product  OutDataType=sfix(16)  OutScaling=2^0  SaturateOnIntegerOverflow=on  RndMeth=Zero  InputSameDT=on  OutDataTypeStr=Inherit: Same as first input
  Sum6 : Sum  Inputs=+-  OutDataType=sfix(16)  OutScaling=2^0  SaturateOnIntegerOverflow=on  InputSameDT=on  OutDataTypeStr=Inherit: Same as first input
  Sum7 : Sum  Inputs=--  OutDataType=sfix(16)  OutScaling=2^0  SaturateOnIntegerOverflow=on  InputSameDT=on  OutDataTypeStr=Inherit: Same as first input
  Sum8 : Sum  OutDataType=sfix(16)  OutScaling=2^0  SaturateOnIntegerOverflow=on  InputSameDT=on  OutDataTypeStr=Inherit: Same as first input
  Sum9 : Sum  Inputs=+-  OutDataType=sfix(16)  OutScaling=2^0  SaturateOnIntegerOverflow=on  InputSameDT=on  OutDataTypeStr=Inherit: Same as first input
  trig : Trigonometry  Operator=cos
  trig1 : Trigonometry
  Cx Cy Cz : Outport  OutDataType=sfix(16)  OutScaling=2^0  InitialOutput=0
  CRb CMb CNb : Outport  Port=2  OutDataType=sfix(16)  OutScaling=2^0  InitialOutput=0
  wires:
  alpha beta alpha_dot beta_dot/1 -> Fcn1/1
  Gain2/1 -> trig/1, trig1/1
  Fcn1/1 -> Gain2/1
  CR CM CN/1 -> Demux2/1
  CL CD CY/1 -> Demux/1
  Mux/1 -> Cx Cy Cz/1
  Product9/1 -> Sum6/1
  Product/1 -> Sum6/2
  Product10/1 -> Sum7/2
  Product11/1 -> Sum7/1
  Demux/1 -> Product9/1, Product11/1
  Demux/2 -> Product/1, Product10/1
  Product13/1 -> Sum8/1
  Product12/1 -> Sum8/2
  Product14/1 -> Sum9/2
  Product15/1 -> Sum9/1
  Demux2/3 -> Product14/1, Product13/1
  Demux2/1 -> Product15/1, Product12/1
  Sum6/1 -> Mux/1
  Sum7/1 -> Mux/3
  Demux/3 -> Mux/2
  Sum9/1 -> Mux1/1
  Sum8/1 -> Mux1/3
  Demux2/2 -> Mux1/2
  Mux1/1 -> CRb CMb CNb/1
  trig1/1 -> Product9/2, Product10/2, Product14/2, Product12/2
  trig/1 -> Product/2, Product11/2, Product15/2, Product13/2

== system gtm_aeromodel/get aero forces and moments/AERODYNAMICS/Aero Incidence Angles/DOWNWASH/deps_hob_ ==
  hob : Inport  OutDataType=sfix(16)  OutScaling=2^0
  alpha : Inport  Port=2  OutDataType=sfix(16)  OutScaling=2^0
  flap : Inport  Port=3  OutDataType=sfix(16)  OutScaling=2^0
  Enable : EnablePort
  depshob_ : Subsystem  mask(1-2-3 Table){@1=depshobx_HOB, @2=depshoby_FALPHA, @3=depshobz_FLPDEF, @4=depshob}
      mask prompts: @1 "X vector:"; @2 "Y vector:"; @3 "Z vector:"; @4 "Table:"
      mask help: 3-D Table Look Up. Enter monotonic X, Y and Z vectors and a matrix of 2-D tables. See the help for more info.
      mask init:
      | x=@1;y=@2;z=@3;tab=@4;
      mask Help: The X, Y and Z vectors must be monotonic.   The 3-D table is a horizontal concatenation of  2-D tables.  X  indexes into the columns of the 2-D tables & Y indexes into the rows of the 2-D tables.  Z indexes into the table levels (starting with the 1st 2-D table).   The input values are x, y and z respectively (e.g., top port = x).
      mask Display: plot([0 2 2 0 0],[0 0 2 2 0],[0 2 2.9 0.95 0],[2 2 2.7 2.7 2],[2 2.9 2.9 2 2],[0 0.85 2.7 2 0])
  depshob : Outport  OutDataType=sfix(16)  OutScaling=2^0  InitialOutput=0
  wires:
  depshob_/1(Interp Value) -> depshob/1
  hob/1 -> depshob_/1(X)
  alpha/1 -> depshob_/2(Y)
  flap/1 -> depshob_/3(Z)

== system gtm_aeromodel/get aero forces and moments/AERODYNAMICS/Aero Incidence Angles/DOWNWASH/depsct ==
  cthrust : Inport  OutDataType=sfix(16)  OutScaling=2^0
  eps_thrust : Product  OutDataType=sfix(16)  OutScaling=2^0  SaturateOnIntegerOverflow=on  RndMeth=Zero  InputSameDT=on  OutDataTypeStr=Inherit: Same as first input
  gbct : Subsystem  mask(1-D Table){z=gbctx_CTTOT, tab=gbct}
      mask prompts: z "Z vector:"; tab "Table:"
      mask help: 1-D Table Look Up. Enter monotonic Z vector amd table. See the help for more info.
      mask Help: The Z vector must be monotonic.  Z indexes into the columns of the 1-D tables.   Table does not extrapolate beyound the break vectors
      mask Display: plot(@2)
  despct : Outport  OutDataType=sfix(16)  OutScaling=2^0  InitialOutput=0
  wires:
  cthrust/1 -> gbct/1(Z), eps_thrust/2
  gbct/1(Interp Value) -> eps_thrust/1
  eps_thrust/1 -> despct/1

== system gtm_aeromodel/get aero forces and moments/AERODYNAMICS/Aero Incidence Angles/DOWNWASH/eps_flap ==
  alpha : Inport  OutDataType=sfix(16)  OutScaling=2^0
  flap : Inport  Port=2  OutDataType=sfix(16)  OutScaling=2^0
  qdyn : Inport  Port=3  OutDataType=sfix(16)  OutScaling=2^0
  flex : Inport  Port=4  OutDataType=sfix(16)  OutScaling=2^0
  Enable : EnablePort
  Product : Product  OutDataType=sfix(16)  OutScaling=2^0  SaturateOnIntegerOverflow=on  RndMeth=Zero  InputSameDT=on  OutDataTypeStr=Inherit: Same as first input
  Sum1 : Sum  Inputs=-+  OutDataType=sfix(16)  OutScaling=2^0  SaturateOnIntegerOverflow=on  InputSameDT=on  OutDataTypeStr=Inherit: Same as first input
  Sum2 : Sum  OutDataType=sfix(16)  OutScaling=2^0  SaturateOnIntegerOverflow=on  InputSameDT=on  OutDataTypeStr=Inherit: Same as first input
  Switch5 : Switch  Threshold=0.5  SaturateOnIntegerOverflow=on  InputSameDT=on
  const : Constant  Value=1.0  OutDataType=sfix(16)  OutScaling=2^0
  dclwbdffr : Subsystem  TreatAsAtomicUnit=on
  eps_spoiler1 : Product  OutDataType=sfix(16)  OutScaling=2^0  SaturateOnIntegerOverflow=on  RndMeth=Zero  InputSameDT=on  OutDataTypeStr=Inherit: Same as first input
  epsa : Subsystem  mask(1-D Table){z=epsax_mach, tab=epsa}
      mask prompts: z "Z vector:"; tab "Table:"
      mask help: 1-D Table Look Up. Enter monotonic Z vector amd table. See the help for more info.
      mask Help: The Z vector must be monotonic.  Z indexes into the columns of the 1-D tables.   Table does not extrapolate beyound the break vectors
      mask Display: plot(@2)
  epsdsbdf : Subsystem  mask(1-2-3 Table){@1=epsdsbdfx_DSB, @2=epsdsbdfy_FALPHA, @3=epsdsbdfz_FLPDEF, @4=epsdsbdf}
      mask prompts: @1 "X vector:"; @2 "Y vector:"; @3 "Z vector:"; @4 "Table:"
      mask help: 3-D Table Look Up. Enter monotonic X, Y and Z vectors and a matrix of 2-D tables. See the help for more info.
      mask init:
      | x=@1;y=@2;z=@3;tab=@4;
      mask Help: The X, Y and Z vectors must be monotonic.   The 3-D table is a horizontal concatenation of  2-D tables.  X  indexes into the columns of the 2-D tables & Y indexes into the rows of the 2-D tables.  Z indexes into the table levels (starting with the 1st 2-D table).   The input values are x, y and z respectively (e.g., top port = x).
      mask Display: plot([0 2 2 0 0],[0 0 2 2 0],[0 2 2.9 0.95 0],[2 2 2.7 2.7 2],[2 2.9 2.9 2 2],[0 0.85 2.7 2 0])
  epsodsb : Subsystem  mask(2-D Table){y=epsodsbx_DSB, z=epsodsby_FMACH, tab=epsodsb}
      mask prompts: y "Y vector:"; z "Z vector:"; tab "Table:"
      mask help: 2-D Table Look Up. Enter monotonic Y and Z vectors and a matrix of 2-D tables. See the help for more info.
      mask Help: The Y and Z vectors must be monotonic.  Y  indexes into the columns of the 2-D table & Z indexes into the rows of the 2-D tables.   The input values are y and z respectively (e.g., top port = y).
      mask Display: plot(-10,-10,110,110,[90,50,10],[90,40,30],[90,50,10],[50,26,20],[90,50,10],[22,13,10])
  mach : Constant  Value=.178  OutDataType=sfix(16)  OutScaling=2^0
  zero : Constant  Value=0  OutDataType=sfix(16)  OutScaling=2^0
  eps_flap : Outport  OutDataType=sfix(16)  OutScaling=2^0  InitialOutput=0
  wires:
  epsodsb/1(Interp Value) -> Sum2/2
  epsdsbdf/1(Interp Value) -> Sum1/2
  Sum1/1 -> Product/1
  epsa/1(Interp Value) -> eps_spoiler1/1
  flex/1 -> dclwbdffr/Enable, Switch5/2
  Switch5/1 -> Product/2
  const/1 -> Switch5/3
  dclwbdffr/1(dclwbdffr) -> Switch5/1
  qdyn/1 -> dclwbdffr/1(qdyn)
  flap/1 -> dclwbdffr/2(flap), epsdsbdf/3(Z)
  zero/1 -> epsdsbdf/1(X), epsodsb/1(Y)
  mach/1 -> epsodsb/2(Z), epsa/1(Z)
  Product/1 -> eps_flap/1
  eps_spoiler1/1 -> Sum2/1
  Sum2/1 -> Sum1/1
  alpha/1 -> epsdsbdf/2(Y), eps_spoiler1/2

== system gtm_aeromodel/get aero forces and moments/AERODYNAMICS/Aero Incidence Angles/DOWNWASH/eps_speedbrake_ ==
  dsb : Inport  OutDataType=sfix(16)  OutScaling=2^0
  mach : Inport  Port=2  OutDataType=sfix(16)  OutScaling=2^0
  Sum1 : Sum  Inputs=-+  OutDataType=sfix(16)  OutScaling=2^0  SaturateOnIntegerOverflow=on  InputSameDT=on  OutDataTypeStr=Inherit: Same as first input
  epsodsb : Subsystem  mask(2-D Table){y=epsodsbx_DSB, z=epsodsby_FMACH, tab=epsodsb}
      mask prompts: y "Y vector:"; z "Z vector:"; tab "Table:"
      mask help: 2-D Table Look Up. Enter monotonic Y and Z vectors and a matrix of 2-D tables. See the help for more info.
      mask Help: The Y and Z vectors must be monotonic.  Y  indexes into the columns of the 2-D table & Z indexes into the rows of the 2-D tables.   The input values are y and z respectively (e.g., top port = y).
      mask Display: plot(-10,-10,110,110,[90,50,10],[90,40,30],[90,50,10],[50,26,20],[90,50,10],[22,13,10])
  epsodsb_0 : Subsystem  mask(2-D Table){y=epsodsbx_DSB, z=epsodsby_FMACH, tab=epsodsb}
      mask prompts: y "Y vector:"; z "Z vector:"; tab "Table:"
      mask help: 2-D Table Look Up. Enter monotonic Y and Z vectors and a matrix of 2-D tables. See the help for more info.
      mask Help: The Y and Z vectors must be monotonic.  Y  indexes into the columns of the 2-D table & Z indexes into the rows of the 2-D tables.   The input values are y and z respectively (e.g., top port = y).
      mask Display: plot(-10,-10,110,110,[90,50,10],[90,40,30],[90,50,10],[50,26,20],[90,50,10],[22,13,10])
  mach1 : Constant  Value=0  OutDataType=sfix(16)  OutScaling=2^0
  deps_sb : Outport  OutDataType=sfix(16)  OutScaling=2^0  InitialOutput=0
  wires:
  Sum1/1 -> deps_sb/1
  epsodsb_0/1(Interp Value) -> Sum1/1
  epsodsb/1(Interp Value) -> Sum1/2
  mach/1 -> epsodsb/2(Z), epsodsb_0/2(Z)
  dsb/1 -> epsodsb/1(Y)
  mach1/1 -> epsodsb_0/1(Y)

== system gtm_aeromodel/get aero forces and moments/AERODYNAMICS/Aero Incidence Angles/DOWNWASH/eps_spoiler_ ==
  dsl : Inport  OutDataType=sfix(16)  OutScaling=2^0
  mach : Inport  Port=2  OutDataType=sfix(16)  OutScaling=2^0
  altitude : Inport  Port=3  OutDataType=sfix(16)  OutScaling=2^0
  flex : Inport  Port=4  OutDataType=sfix(16)  OutScaling=2^0
  dsb : Inport  Port=5  OutDataType=sfix(16)  OutScaling=2^0
  dsr : Inport  Port=6  OutDataType=sfix(16)  OutScaling=2^0
  Sum1 : Sum  OutDataType=sfix(16)  OutScaling=2^0  SaturateOnIntegerOverflow=on  InputSameDT=on  OutDataTypeStr=Inherit: Same as first input
  Sum2 : Sum  Inputs=+-  OutDataType=sfix(16)  OutScaling=2^0  SaturateOnIntegerOverflow=on  InputSameDT=on  OutDataTypeStr=Inherit: Same as first input
  Sum3 : Sum  Inputs=+-  OutDataType=sfix(16)  OutScaling=2^0  SaturateOnIntegerOverflow=on  InputSameDT=on  OutDataTypeStr=Inherit: Same as first input
  Switch5 : Switch  Threshold=0.5  SaturateOnIntegerOverflow=on  InputSameDT=on
  const : Constant  Value=1.0  OutDataType=sfix(16)  OutScaling=2^0
  dclsbfr_ : Subsystem  TreatAsAtomicUnit=on
  epsodsl : Subsystem  mask(2-D Table){y=epsodslx_DSL, z=epsodsly_FMACH, tab=epsodsl}
      mask prompts: y "Y vector:"; z "Z vector:"; tab "Table:"
      mask help: 2-D Table Look Up. Enter monotonic Y and Z vectors and a matrix of 2-D tables. See the help for more info.
      mask Help: The Y and Z vectors must be monotonic.  Y  indexes into the columns of the 2-D table & Z indexes into the rows of the 2-D tables.   The input values are y and z respectively (e.g., top port = y).
      mask Display: plot(-10,-10,110,110,[90,50,10],[90,40,30],[90,50,10],[50,26,20],[90,50,10],[22,13,10])
  epsodsl_ : Subsystem  mask(2-D Table){y=epsodslx_DSL, z=epsodsly_FMACH, tab=epsodsl}
      mask prompts: y "Y vector:"; z "Z vector:"; tab "Table:"
      mask help: 2-D Table Look Up. Enter monotonic Y and Z vectors and a matrix of 2-D tables. See the help for more info.
      mask Help: The Y and Z vectors must be monotonic.  Y  indexes into the columns of the 2-D table & Z indexes into the rows of the 2-D tables.   The input values are y and z respectively (e.g., top port = y).
      mask Display: plot(-10,-10,110,110,[90,50,10],[90,40,30],[90,50,10],[50,26,20],[90,50,10],[22,13,10])
  epsodsl_1 : Subsystem  mask(2-D Table){y=epsodslx_DSL, z=epsodsly_FMACH, tab=epsodsl}
      mask prompts: y "Y vector:"; z "Z vector:"; tab "Table:"
      mask help: 2-D Table Look Up. Enter monotonic Y and Z vectors and a matrix of 2-D tables. See the help for more info.
      mask Help: The Y and Z vectors must be monotonic.  Y  indexes into the columns of the 2-D table & Z indexes into the rows of the 2-D tables.   The input values are y and z respectively (e.g., top port = y).
      mask Display: plot(-10,-10,110,110,[90,50,10],[90,40,30],[90,50,10],[50,26,20],[90,50,10],[22,13,10])
  epsodsl_2 : Subsystem  mask(2-D Table){y=epsodslx_DSL, z=epsodsly_FMACH, tab=epsodsl}
      mask prompts: y "Y vector:"; z "Z vector:"; tab "Table:"
      mask help: 2-D Table Look Up. Enter monotonic Y and Z vectors and a matrix of 2-D tables. See the help for more info.
      mask Help: The Y and Z vectors must be monotonic.  Y  indexes into the columns of the 2-D table & Z indexes into the rows of the 2-D tables.   The input values are y and z respectively (e.g., top port = y).
      mask Display: plot(-10,-10,110,110,[90,50,10],[90,40,30],[90,50,10],[50,26,20],[90,50,10],[22,13,10])
  deps_sp : Outport  OutDataType=sfix(16)  OutScaling=2^0  InitialOutput=0
  dclsbfr : Outport  Port=2  OutDataType=sfix(16)  OutScaling=2^0  InitialOutput=0
  wires:
  Sum1/1 -> deps_sp/1
  mach/1 -> epsodsl/2(Z), epsodsl_/2(Z), dclsbfr_/2(mach), epsodsl_2/2(Z), epsodsl_1/2(Z)
  epsodsl/1(Interp Value) -> Sum2/1
  dsr/1 -> epsodsl_1/1(Y)
  epsodsl_1/1(Interp Value) -> Sum3/1
  Switch5/1 -> dclsbfr/1
  flex/1 -> dclsbfr_/Enable, Switch5/2
  dclsbfr_/1(dclsbfr) -> Switch5/1
  const/1 -> Switch5/3
  altitude/1 -> dclsbfr_/1(altitude)
  epsodsl_/1(Interp Value) -> Sum2/2
  epsodsl_2/1(Interp Value) -> Sum3/2
  dsb/1 -> epsodsl_/1(Y), epsodsl_2/1(Y)
  dsl/1 -> epsodsl/1(Y)
  Sum2/1 -> Sum1/1
  Sum3/1 -> Sum1/2
